simulink model "xy_table"  (R2020b)
settings: Solver=VariableStepAuto  StartTime=0.0  StopTime=2  RelTol=1e-3
undefined symbols (not defined in the file): B_x, B_y, J_ex, J_ey, K_a, K_e, K_t, T_i
libraries: cstblocks x2, simulink x1
settings Model: Creator=jasper  LastModifiedBy=jasper

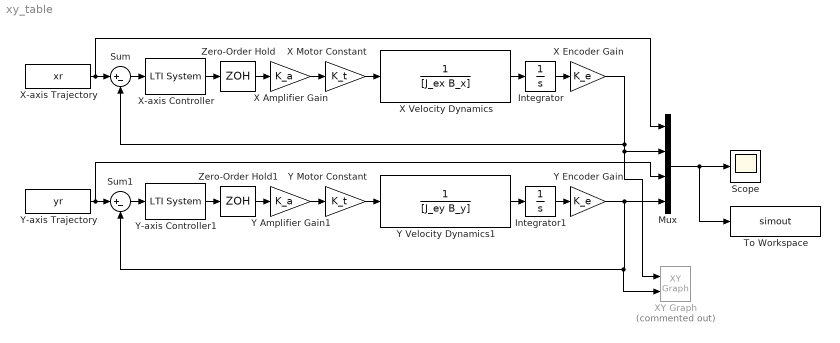
== system xy_table ==
  Integrator : Integrator
  Integrator1 : Integrator
  Mux : Mux
  Scope : Scope
  Sum : Sum  Inputs=|+-
  Sum1 : Sum  Inputs=|+-
  To Workspace : ToWorkspace  VariableName=simout  SaveFormat=Timeseries  SampleTime=-1
  X Amplifier Gain : Gain  Gain=K_a
  X Encoder Gain : Gain  Gain=K_e
  X Motor Constant : Gain  Gain=K_t
  X Velocity Dynamics : TransferFcn  Denominator=[J_ex B_x]
  X-axis Controller : cstblocks/LTI System  sys=contx_z  IC=[]
  X-axis Trajectory : FromWorkspace  VariableName=xr
  XY Graph : simulink/Sinks/XY Graph  Commented=on  xmin=-1  xmax=1  ymin=-1  ymax=1  st=-1
  Y Amplifier Gain1 : Gain  Gain=K_a
  Y Encoder Gain : Gain  Gain=K_e
  Y Motor Constant : Gain  Gain=K_t
  Y Velocity Dynamics1 : TransferFcn  Denominator=[J_ey B_y]
  Y-axis Controller1 : cstblocks/LTI System  sys=conty_z  IC=[]
  Y-axis Trajectory : FromWorkspace  VariableName=yr
  Zero-Order Hold : ZeroOrderHold  SampleTime=T_i
  Zero-Order Hold1 : ZeroOrderHold  SampleTime=T_i
  wires:
  X-axis Trajectory/1 -> Mux/1, Sum/1
  Sum/1 -> X-axis Controller/1
  X-axis Controller/1 -> Zero-Order Hold/1
  Zero-Order Hold/1 -> X Amplifier Gain/1
  X Amplifier Gain/1 -> X Motor Constant/1
  X Motor Constant/1 -> X Velocity Dynamics/1
  X Velocity Dynamics/1 -> Integrator/1
  Integrator/1 -> X Encoder Gain/1
  X Encoder Gain/1 -> Mux/2, XY Graph/1, Sum/2
  Y-axis Controller1/1 -> Zero-Order Hold1/1
  Y Encoder Gain/1 -> Mux/4, XY Graph/2, Sum1/2
  Y-axis Trajectory/1 -> Mux/3, Sum1/1
  Integrator1/1 -> Y Encoder Gain/1
  Zero-Order Hold1/1 -> Y Amplifier Gain1/1
  Y Velocity Dynamics1/1 -> Integrator1/1
  Y Amplifier Gain1/1 -> Y Motor Constant/1
  Y Motor Constant/1 -> Y Velocity Dynamics1/1
  Sum1/1 -> Y-axis Controller1/1
  Mux/1 -> To Workspace/1, Scope/1
